simulink model "AircraftModel"  (R2021b)
settings: Solver=VariableStepAuto  StartTime=0.0  StopTime=simTim  RelTol=1e-3
values from neighbouring files (symbols this model uses):
  deltaA = inputs(3)    [FlatEarthEquations.m]    (also in RunAircraftModel.m = 0)
  deltaE = inputs(4)    [FlatEarthEquations.m]    (also in RunAircraftModel.m = -0.100000035756)
  deltaR = inputs(5)    [FlatEarthEquations.m]    (also in RunAircraftModel.m = 0)
  deltaT1 = inputs(1)    [FlatEarthEquations.m]    (also in RunAircraftModel.m = 0.0799999936985)
  deltaT2 = inputs(2)    [FlatEarthEquations.m]    (also in RunAircraftModel.m = 0.0799999936985)
  X0 = [pN0; pE0; h0; phi0; theta0; psi0; U0; V0; W0; P0; Q0; R0]    [RunAircraftModel.m]
undefined symbols (not defined in the file or in its folder): FlatEarthEquations
settings Model: Creator=Reza  LastModifiedBy=mo112

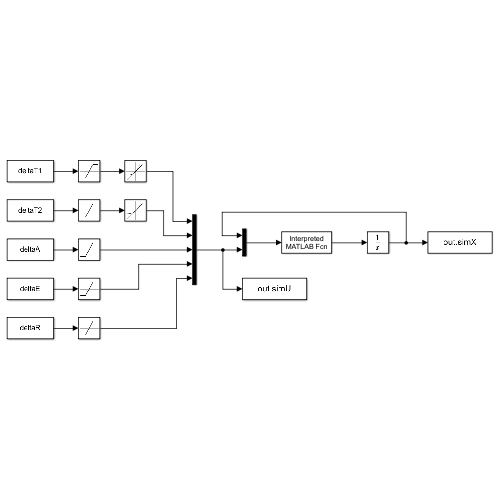
[thumbnail: Simulink's stored preview of the top-level diagram]
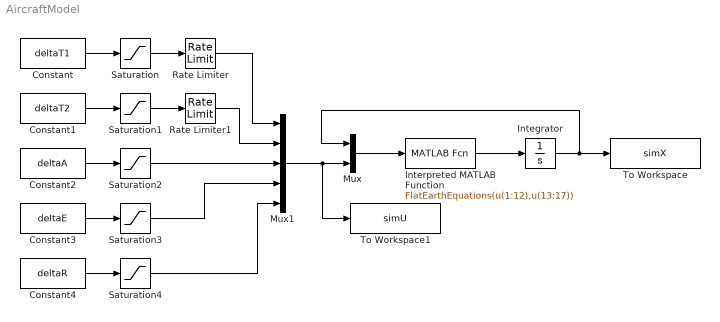
== system AircraftModel ==
  Constant : Constant  Value=deltaT1
  Constant1 : Constant  Value=deltaT2
  Constant2 : Constant  Value=deltaA
  Constant3 : Constant  Value=deltaE
  Constant4 : Constant  Value=deltaR
  Integrator : Integrator  InitialCondition=X0
  Interpreted MATLAB Function : MATLABFcn  MATLABFcn=FlatEarthEquations(u(1:12),u(13:17))
  Mux : Mux  Inputs=2
  Mux1 : Mux  Inputs=5
  Rate Limiter : RateLimiter  RisingSlewLimit=1.6  FallingSlewLimit=-1.6  SampleTimeMode=inherited
  Rate Limiter1 : RateLimiter  RisingSlewLimit=1.6  FallingSlewLimit=-1.6  SampleTimeMode=inherited
  Saturation : Saturate  UpperLimit=1*pi/180  LowerLimit=0.5*pi/180
  Saturation1 : Saturate  UpperLimit=1*pi/180  LowerLimit=0.5*pi/180
  Saturation2 : Saturate  UpperLimit=25*pi/180  LowerLimit=-25*pi/180
  Saturation3 : Saturate  UpperLimit=10*pi/180  LowerLimit=-25*pi/180
  Saturation4 : Saturate  UpperLimit=30*pi/180  LowerLimit=-30*pi/180
  To Workspace : ToWorkspace  VariableName=simX  SaveFormat=Timeseries  SampleTime=-1
  To Workspace1 : ToWorkspace  VariableName=simU  SaveFormat=Timeseries  SampleTime=-1
  wires:
  Interpreted MATLAB Function/1 -> Integrator/1
  Mux/1 -> Interpreted MATLAB Function/1
  Integrator/1 -> To Workspace/1, Mux/1
  Rate Limiter/1 -> Mux1/1
  Rate Limiter1/1 -> Mux1/2
  Saturation/1 -> Rate Limiter/1
  Saturation1/1 -> Rate Limiter1/1
  Constant/1 -> Saturation/1
  Constant1/1 -> Saturation1/1
  Constant2/1 -> Saturation2/1
  Constant3/1 -> Saturation3/1
  Constant4/1 -> Saturation4/1
  Mux1/1 -> To Workspace1/1, Mux/2
  Saturation2/1 -> Mux1/3
  Saturation3/1 -> Mux1/4
  Saturation4/1 -> Mux1/5
